simulink model "foc_signum_smo_g4"  (R2021b)
settings: Solver=FixedStepDiscrete  StartTime=0.0  StopTime=6  FixedStep=Tsw  RelTol=1e-3
undefined symbols (not defined in the file): a, B, b, current_ki, current_kp, DiscIntNeverNeededParam, Ibase, id_ref, J, k1_sta, k2_sta, Ks, load_torque, Ls, qpll, Rs, sigmoid_a, speed_ki, speed_kp, Ts_speed, Tsw, Vbase, Vdc, wbase
libraries: mcbcontrolslib x6, mcbplantlib x1, autolibpmsmexterior x1, simulink_extras x1
settings Model: Creator=gary  LastModifiedBy=gary
settings DebuggingCC: SFMachineParentedDataDiag=warning

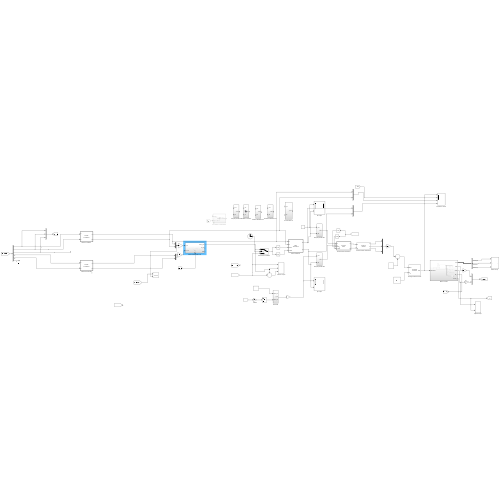
[thumbnail: Simulink's stored preview of the top-level diagram]
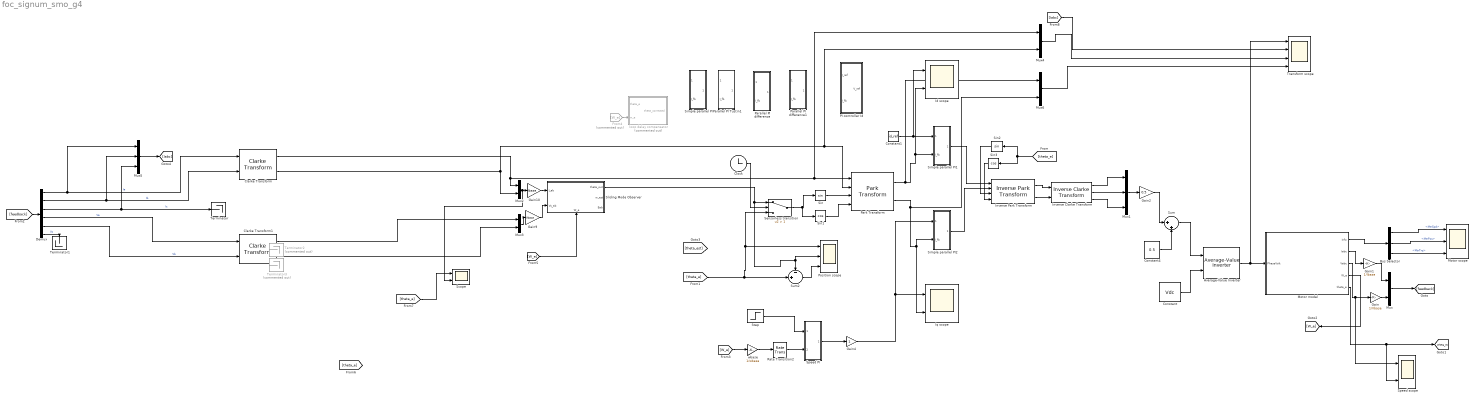
== system foc_signum_smo_g4 ==
  Average-Value Inverter : mcbplantlib/Average-Value Inverter
  Bus Selector : BusSelector  OutputSignals=MtrSpd,MtrPos,MtrTrq
  Clarke Transform : mcbcontrolslib/Clarke Transform  VariantControl=Variant2
  Clarke Transform1 : mcbcontrolslib/Clarke Transform  VariantControl=Variant2
  Clock : Clock
  Constant : Constant  Value=Vdc
  Constant1 : Constant  Value=id_ref
  Constant4 : Constant  Value=0.5
  Demux : Demux  Outputs=6
  From4 : From  Commented=on  GotoTag=W_e
  Gain : Gain  Gain=1/Vbase
  Gain1 : Gain  Gain=1/Ibase
  Gain10 : Gain  Gain=Ibase
  Gain2 : Gain  Gain=0.5
  Gain4 : Gain
  Gain9 : Gain  Gain=Vbase
  Id scope : Scope  NumInputPorts=2
  Inverse Clarke Transform : mcbcontrolslib/Inverse Clarke Transform
      settings: SourceProductBaseCode=MT
  Inverse Park Transform : mcbcontrolslib/Inverse Park Transform  AxisAlignment=D-axis
  Iq scope : Scope  NumInputPorts=2
  Motor model : Subsystem
  Motor scope : Scope  NumInputPorts=3
  Mux{,2..4,6} (5 alike) : Mux  Inputs=2
  Mux1 : Mux  Inputs=3
  Mux5 : Mux  Inputs=3
  PI controller Id : Subsystem
  Parallel PI Tustin1 : Subsystem
  Parallel PI difference : Subsystem
  Parallel PI difference1 : Subsystem
  Park Transform : mcbcontrolslib/Park Transform  AxisAlignment=D-axis
      settings: SourceProductBaseCode=MT
  Position scope : Scope  NumInputPorts=3
  Rate Transition2 : RateTransition  OutPortSampleTime=Ts_speed
  Scope : Scope  NumInputPorts=2
  Sensorless transition : Switch  Criteria=u2 > Threshold  Threshold=1
  Simple parallel PI : Subsystem
  Simple parallel PI1 : Subsystem
  Simple parallel PI2 : Subsystem
  Sin : Trigonometry
  Sin1 : Trigonometry  Operator=cos
  Sin2 : Trigonometry
  Sin3 : Trigonometry  Operator=cos
  Sliding Mode Observer : Subsystem
      settings: PortSchema="{\"entries\":[{\"content\":{\"sides\":[{\"content\":{\"connectorIds\":[\"In1\",\"In2\"]},\"type\":\"ConnectorPlacement.EquallySpacedRectSide\",\"uuid\":\"577b0a5e-906f-48ed-8129-dbceeacd07ca\"},{\"content\":{\"connectorIds\":[\"Out1\",\"Out2\",\"Out3\"],\"side\":\"RIGHT\"},\"type\":\"ConnectorPlacement.EquallySpacedRectSide\",\"uuid\":\"748cd512-9e16-4867-9350-2ceae49fd380\"},{\"content\":{\"connectorIds\":[],\"side\":\"TOP\"},\"type\":\"ConnectorPlacement.EquallySpacedRectSide\",\"uuid\":\"9a069db4-944b-4d2f-847d-3587eda2386e\"},{\"content\":{\"connectorIds\":[\"In3\"],\"side\":\"BOTTOM\"},\"type\":\"ConnectorPlacement.EquallySpacedRectSide\",\"uuid\":\"f06943a4-3386-47cc-a738-6805519a12d9\"}]},\"type\":\"ConnectorPlacement.EquallySpacedConnector\",\"uuid\":\"48fa9e95-782d-48ca-a522-50122ca51ecb\"}],\"packageUris\":[\"http://schema.mathworks.com/mf0/Connector/R2020b\"],\"version\":\"1.0\"}"
  Speed PI : Subsystem
  Speed scope : Scope  NumInputPorts=2
  Step : Step  Time=3  Before=0.25  After=0.5  SampleTime=0
  Sum : Sum  Inputs=|++
  Sum2 : Sum  Inputs=-+|
  Terminator : Terminator
  Terminator1 : Terminator
  Terminator2 : Terminator  Commented=on
  Terminator3 : Terminator  Commented=on
  Transform scope : Scope  NumInputPorts=4
  loop delay compensator : Subsystem  Commented=on
  wbase : Gain  Gain=1/wbase
  wires:
  Constant/1 -> Average-Value Inverter/2
  Motor model/1(Info) -> Bus Selector/1
  Bus Selector/2 -> Motor scope/2  "<MtrPos>"
  Bus Selector/3 -> Motor scope/3  "<MtrTrq>"
  Mux/1 -> [feedback]
  [feedback] -> Demux/1
  Demux/3 -> Mux5/3, Terminator/1  "Ic"
  Demux/1 -> Mux5/1, Clarke Transform/1  "Ia"
  Demux/2 -> Mux5/2, Clarke Transform/2  "Ib"
  Park Transform/1 -> Simple parallel PI1/2(I_fb), Id scope/2, Mux6/1
  Park Transform/2 -> Mux6/2, Simple parallel PI2/2(I_fb), Iq scope/2
  Constant1/1 -> Simple parallel PI1/1(I_ref), Id scope/1
  Simple parallel PI1/1(Vref) -> Inverse Park Transform/1
  Simple parallel PI2/1(Vref) -> Inverse Park Transform/2
  Inverse Park Transform/1 -> Inverse Clarke Transform/1
  Inverse Park Transform/2 -> Inverse Clarke Transform/2
  Inverse Clarke Transform/2 -> Mux1/2
  Inverse Clarke Transform/3 -> Mux1/3
  Inverse Clarke Transform/1 -> Mux1/1
  Motor model/2(Iabc) -> Gain1/1
  Gain1/1 -> Mux/1
  Motor model/3(Vabc) -> Speed scope/1, Gain/1
  Demux/6 -> Terminator1/1  "Vc"
  Clarke Transform/1 -> Mux2/1, Mux4/1, Park Transform/1
  Clarke Transform/2 -> Mux2/2, Mux4/2, Park Transform/2
  Sin/1 -> Park Transform/3
  Sin1/1 -> Park Transform/4
  Gain/1 -> Mux/2
  Mux1/1 -> Gain2/1
  Gain2/1 -> Sum/1
  Sum/1 -> Average-Value Inverter/1
  Constant4/1 -> Sum/2
  [theta_e] -> Position scope/1, Sensorless transition/3, Sum2/2
  Bus Selector/1 -> Motor scope/1  "<MtrSpd>"
  Clock/1 -> Sensorless transition/2
  Sliding Mode Observer/1(theta_out) -> Sum2/1, Position scope/2, Sensorless transition/1
  [W_e] -> wbase/1
  Step/1 -> Speed PI/1(Speed_ref)
  Rate Transition2/1 -> Speed PI/2(Speed_fb)
  Speed PI/1(I_ref) -> Gain4/1
  wbase/1 -> Rate Transition2/1
  Motor model/4(W_e) -> [W_e]
  Gain4/1 -> Simple parallel PI2/1(I_ref), Iq scope/1
  Demux/4 -> Clarke Transform1/1  "Va"
  Demux/5 -> Clarke Transform1/2  "Vb"
  Mux2/1 -> Scope/2, Gain10/1
  Gain10/1 -> Sliding Mode Observer/1(I_ab)
  Mux3/1 -> Gain9/1
  Gain9/1 -> Sliding Mode Observer/2(Vs_ab)
  Sum2/1 -> Position scope/3
  Clarke Transform1/1 -> Mux3/1
  Clarke Transform1/2 -> Mux3/2
  Average-Value Inverter/1 -> Transform scope/1, Motor model/1(PhaseVolt)
  From4/1 -> loop delay compensator/2(w_e)
  Sin2/1 -> Inverse Park Transform/3
  Sin3/1 -> Inverse Park Transform/4
  [theta_e] -> Sin2/1, Sin3/1
  Mux4/1 -> Transform scope/3
  Mux6/1 -> Transform scope/4
  Mux5/1 -> [Iabc]
  [Iabc] -> Transform scope/2
  [W_e] -> Sliding Mode Observer/3(W_e)
  Sensorless transition/1 -> Sin1/1, Sin/1
  Motor model/5(theta_e) -> Speed scope/2, [theta_e]
  [theta_e] -> Scope/1

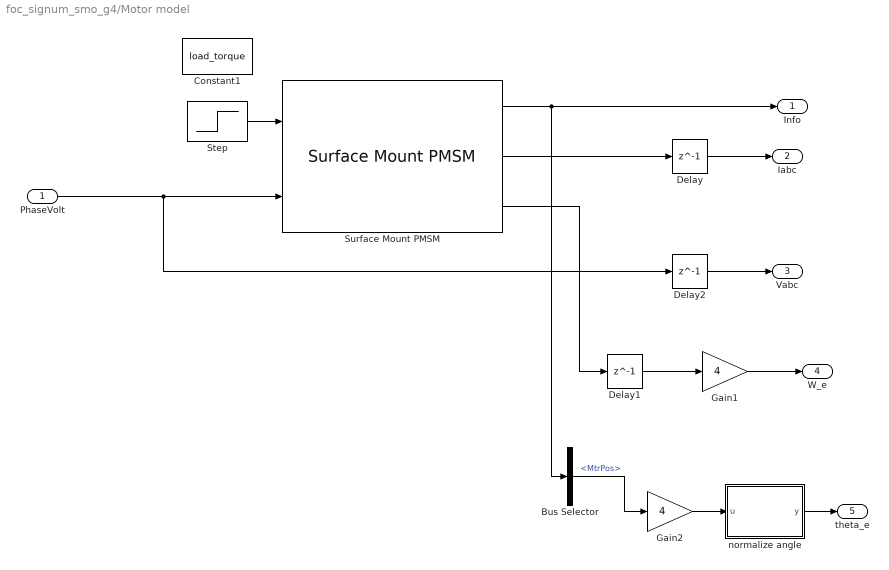
== system foc_signum_smo_g4/Motor model ==
  PhaseVolt : Inport
  Bus Selector : BusSelector  OutputSignals=MtrPos
  Constant1 : Constant  Value=load_torque
  Delay : Delay  DelayLength=1  InitialCondition=0
  Delay1 : Delay  DelayLength=1  InitialCondition=0
  Delay2 : Delay  DelayLength=1  InitialCondition=0
  Gain1 : Gain  Gain=4
  Gain2 : Gain  Gain=4
  Step : Step  Time=4  Before=-0.2  After=-0.4  SampleTime=0
  Surface Mount PMSM : autolibpmsmexterior/Surface Mount PMSM  port_config=Torque  sim_type=Discrete  Ts=Tsw  P=4  Rs=1.5*Rs  Ldq_=2*Ls  KConstText=Permanent flux linkage constant (lambda_pm):  lambda_pm=lambda  Ke=159.9771  Kt=1.323  mechanical=[J, B, 0]  idq0=[0 0]  theta_init=0  omega_init=150  KConst=lambda  lambda_pm_calc=lambda  RefBlkName='autolibpmsmexterior/Surface Mount PMSM'  aMode=5  Ldq="[0.0017      0.0017]"
      settings: SourceProductBaseCode=PW,DR,MT,UV,VE
  normalize angle : MATLAB Function  TreatAsAtomicUnit=on
  Info : Outport
  Iabc : Outport  Port=2
  Vabc : Outport  Port=3
  W_e : Outport  Port=4
  theta_e : Outport  Port=5
  wires:
  Surface Mount PMSM/1 -> Info/1, Bus Selector/1
  Surface Mount PMSM/2 -> Delay/1
  PhaseVolt/1 -> Delay2/1, Surface Mount PMSM/2
  Step/1 -> Surface Mount PMSM/1
  Surface Mount PMSM/3 -> Delay1/1
  Delay/1 -> Iabc/1
  Bus Selector/1 -> Gain2/1  "<MtrPos>"
  Delay1/1 -> Gain1/1
  Gain1/1 -> W_e/1
  Delay2/1 -> Vabc/1
  Gain2/1 -> normalize angle/1(u)
  normalize angle/1(y) -> theta_e/1

== system foc_signum_smo_g4/PI controller Id ==
  I_ref : Inport
  I_fb : Inport  Port=2
  Constant1 : Constant  Value=0
  Constant2 : Constant  Value=current_kp
  Constant3 : Constant  Value=current_ki*Tsw
  Constant4 : Constant  Value=0
  Discrete PI Controller with anti-windup & reset : mcbcontrolslib/Discrete PI Controller  with anti-windup & reset  UpperSaturationLimit=1  LowerSaturationLimit=-1
      settings: SourceProductBaseCode=MT
  Sum : Sum  Inputs=|+-
  V_ref : Outport
  wires:
  I_ref/1 -> Sum/1
  Constant4/1 -> Discrete PI Controller with anti-windup & reset/5
  Discrete PI Controller with anti-windup & reset/1 -> V_ref/1
  Constant1/1 -> Discrete PI Controller with anti-windup & reset/4
  I_fb/1 -> Sum/2
  Constant2/1 -> Discrete PI Controller with anti-windup & reset/2
  Sum/1 -> Discrete PI Controller with anti-windup & reset/1
  Constant3/1 -> Discrete PI Controller with anti-windup & reset/3

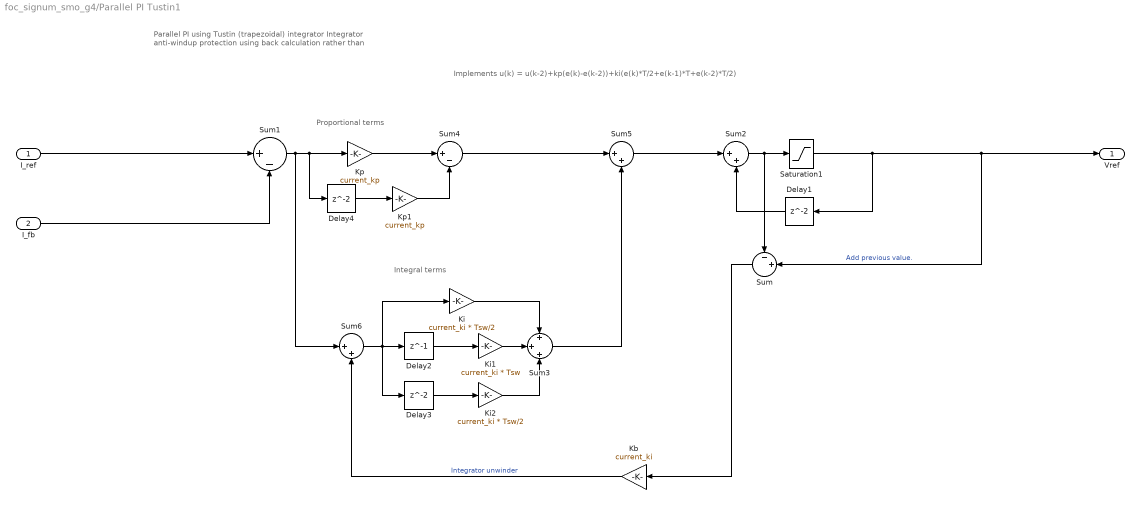
== system foc_signum_smo_g4/Parallel PI Tustin1 ==
  note: Implements u(k) = u(k-2)+kp(e(k)-e(k-2))+ki(e(k)*T/2+e(k-1)*T+e(k-2)*T/2)
  note: Integral terms
  note: Proportional terms
  note: Parallel PI using Tustin (trapezoidal) integrator
      | Integrator anti-windup protection using back calculation
      | rather than
  I_ref : Inport
  I_fb : Inport  Port=2
  Delay1 : Delay  InitialCondition=0
  Delay2 : Delay  DelayLength=1  InitialCondition=0
  Delay3 : Delay  InitialCondition=0
  Delay4 : Delay  InitialCondition=0
  Kb : Gain  Gain=current_ki
  Ki : Gain  Gain=current_ki * Tsw/2
  Ki1 : Gain  Gain=current_ki * Tsw
  Ki2 : Gain  Gain=current_ki * Tsw/2
  Kp : Gain  Gain=current_kp
  Kp1 : Gain  Gain=current_kp
  Saturation1 : Saturate  UpperLimit=1  LowerLimit=-1
  Sum : Sum  Inputs=-+|
  Sum1 : Sum  Inputs=|+-
  Sum2 : Sum  Inputs=|++
  Sum3 : Sum  Inputs=+|+|+
  Sum4 : Sum  Inputs=|+-
  Sum5 : Sum  Inputs=|++
  Sum6 : Sum  Inputs=|++
  Vref : Outport
  wires:
  Sum1/1 -> Sum6/1, Delay4/1, Kp/1
  I_fb/1 -> Sum1/2
  I_ref/1 -> Sum1/1
  Kp/1 -> Sum4/1
  Delay1/1 -> Sum2/2
  Sum2/1 -> Sum/1, Saturation1/1
  Sum/1 -> Kb/1
  Delay2/1 -> Ki1/1
  Delay3/1 -> Ki2/1
  Delay4/1 -> Kp1/1
  Kp1/1 -> Sum4/2
  Ki1/1 -> Sum3/2
  Ki/1 -> Sum3/1
  Ki2/1 -> Sum3/3
  Sum4/1 -> Sum5/1
  Sum6/1 -> Delay3/1, Delay2/1, Ki/1
  Sum3/1 -> Sum5/2
  Sum5/1 -> Sum2/1
  Kb/1 -> Sum6/2  "Integrator unwinder"
  Saturation1/1 -> Sum/2, Vref/1, Delay1/1  "Add previous value."

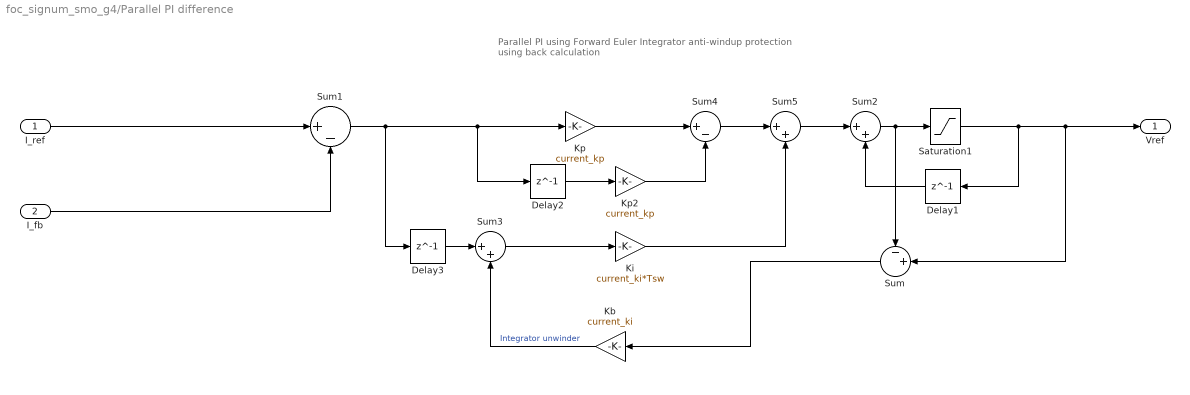
== system foc_signum_smo_g4/Parallel PI difference ==
  note: Parallel PI using Forward Euler
      | Integrator anti-windup protection using back calculation
  I_ref : Inport
  I_fb : Inport  Port=2
  Delay1 : Delay  DelayLength=1  InitialCondition=0
  Delay2 : Delay  DelayLength=1  InitialCondition=0
  Delay3 : Delay  DelayLength=1  InitialCondition=0
  Kb : Gain  Gain=current_ki
  Ki : Gain  Gain=current_ki*Tsw
  Kp : Gain  Gain=current_kp
  Kp2 : Gain  Gain=current_kp
  Saturation1 : Saturate  UpperLimit=1  LowerLimit=0
  Sum : Sum  Inputs=-+|
  Sum1 : Sum  Inputs=|+-
  Sum2 : Sum  Inputs=|++
  Sum3 : Sum  Inputs=|++
  Sum4 : Sum  Inputs=|+-
  Sum5 : Sum  Inputs=|++
  Vref : Outport
  wires:
  I_fb/1 -> Sum1/2
  I_ref/1 -> Sum1/1
  Sum1/1 -> Delay2/1, Kp/1, Delay3/1
  Kp/1 -> Sum4/1
  Delay1/1 -> Sum2/2
  Sum2/1 -> Saturation1/1, Sum/1
  Saturation1/1 -> Sum/2, Vref/1, Delay1/1
  Kb/1 -> Sum3/2  "Integrator unwinder"
  Sum/1 -> Kb/1
  Delay2/1 -> Kp2/1
  Kp2/1 -> Sum4/2
  Sum3/1 -> Ki/1
  Delay3/1 -> Sum3/1
  Sum4/1 -> Sum5/1
  Ki/1 -> Sum5/2
  Sum5/1 -> Sum2/1

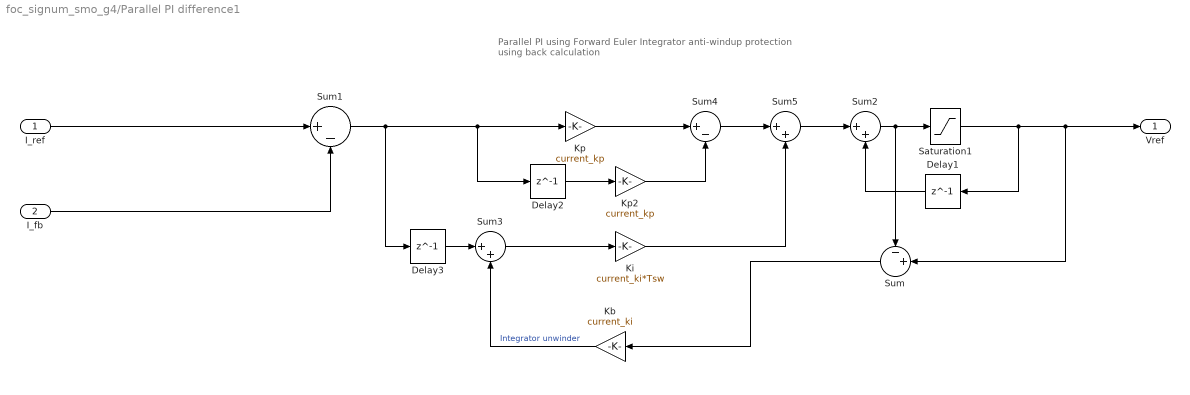
== system foc_signum_smo_g4/Parallel PI difference1 ==
  note: Parallel PI using Forward Euler
      | Integrator anti-windup protection using back calculation
  I_ref : Inport
  I_fb : Inport  Port=2
  Delay1 : Delay  DelayLength=1  InitialCondition=0
  Delay2 : Delay  DelayLength=1  InitialCondition=0
  Delay3 : Delay  DelayLength=1  InitialCondition=0
  Kb : Gain  Gain=current_ki
  Ki : Gain  Gain=current_ki*Tsw
  Kp : Gain  Gain=current_kp
  Kp2 : Gain  Gain=current_kp
  Saturation1 : Saturate  UpperLimit=1  LowerLimit=0
  Sum : Sum  Inputs=-+|
  Sum1 : Sum  Inputs=|+-
  Sum2 : Sum  Inputs=|++
  Sum3 : Sum  Inputs=|++
  Sum4 : Sum  Inputs=|+-
  Sum5 : Sum  Inputs=|++
  Vref : Outport
  wires:
  I_fb/1 -> Sum1/2
  I_ref/1 -> Sum1/1
  Sum1/1 -> Delay2/1, Kp/1, Delay3/1
  Kp/1 -> Sum4/1
  Delay1/1 -> Sum2/2
  Sum2/1 -> Saturation1/1, Sum/1
  Saturation1/1 -> Sum/2, Vref/1, Delay1/1
  Kb/1 -> Sum3/2  "Integrator unwinder"
  Sum/1 -> Kb/1
  Delay2/1 -> Kp2/1
  Kp2/1 -> Sum4/2
  Sum3/1 -> Ki/1
  Delay3/1 -> Sum3/1
  Sum4/1 -> Sum5/1
  Ki/1 -> Sum5/2
  Sum5/1 -> Sum2/1

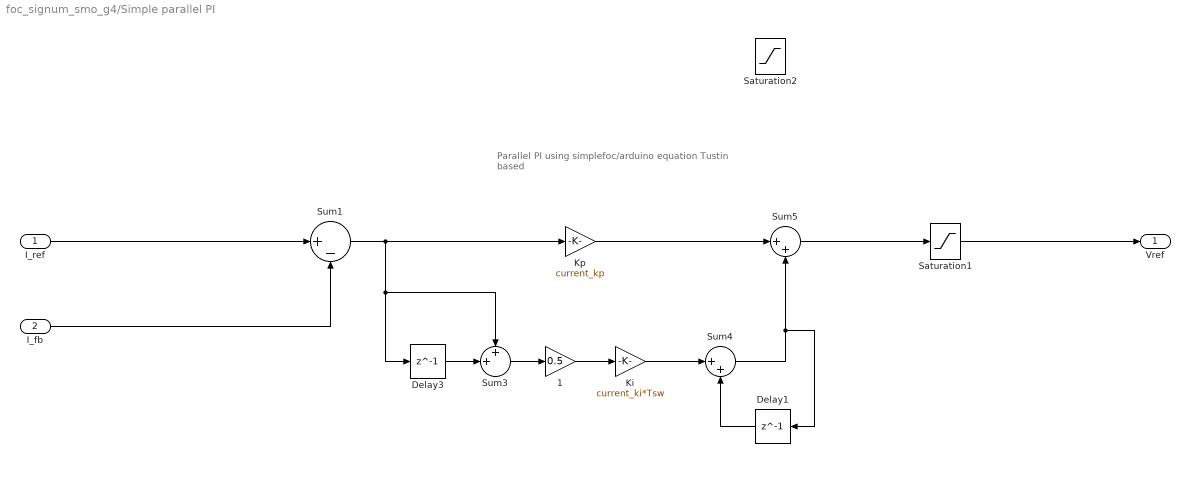
== system foc_signum_smo_g4/Simple parallel PI ==
  note: Parallel PI using simplefoc/arduino equation
      | Tustin based
  I_ref : Inport
  I_fb : Inport  Port=2
  1 : Gain  Gain=0.5
  Delay1 : Delay  DelayLength=1  InitialCondition=0
  Delay3 : Delay  DelayLength=1  InitialCondition=0
  Ki : Gain  Gain=current_ki*Tsw
  Kp : Gain  Gain=current_kp
  Saturation1 : Saturate  UpperLimit=1  LowerLimit=0
  Saturation2 : Saturate  UpperLimit=1  LowerLimit=0
  Sum1 : Sum  Inputs=|+-
  Sum3 : Sum  Inputs=++|
  Sum4 : Sum  Inputs=|++
  Sum5 : Sum  Inputs=|++
  Vref : Outport
  wires:
  I_fb/1 -> Sum1/2
  I_ref/1 -> Sum1/1
  Sum5/1 -> Saturation1/1
  Saturation1/1 -> Vref/1
  Sum3/1 -> 1/1
  Kp/1 -> Sum5/1
  Delay3/1 -> Sum3/2
  Sum1/1 -> Kp/1, Sum3/1, Delay3/1
  1/1 -> Ki/1
  Ki/1 -> Sum4/1
  Sum4/1 -> Delay1/1, Sum5/2
  Delay1/1 -> Sum4/2

== system foc_signum_smo_g4/Simple parallel PI1 ==
  note: Parallel PI using simplefoc/arduino equation
      | Tustin based
  I_ref : Inport
  I_fb : Inport  Port=2
  1 : Gain  Gain=0.5
  Delay1 : Delay  DelayLength=1  InitialCondition=0
  Delay3 : Delay  DelayLength=1  InitialCondition=0
  Ki : Gain  Gain=current_ki*Tsw
  Kp : Gain  Gain=current_kp
  Saturation1 : Saturate  UpperLimit=1  LowerLimit=-1
  Saturation2 : Saturate  UpperLimit=1  LowerLimit=0
  Sum1 : Sum  Inputs=|+-
  Sum3 : Sum  Inputs=++|
  Sum4 : Sum  Inputs=|++
  Sum5 : Sum  Inputs=|++
  Vref : Outport
  wires:
  I_fb/1 -> Sum1/2
  I_ref/1 -> Sum1/1
  Sum5/1 -> Saturation1/1
  Saturation1/1 -> Vref/1
  Sum3/1 -> 1/1
  Kp/1 -> Sum5/1
  Delay3/1 -> Sum3/2
  Sum1/1 -> Kp/1, Sum3/1, Delay3/1
  1/1 -> Ki/1
  Ki/1 -> Sum4/1
  Sum4/1 -> Delay1/1, Sum5/2
  Delay1/1 -> Sum4/2

== system foc_signum_smo_g4/Simple parallel PI2 ==
  note: Parallel PI using simplefoc/arduino equation
      | Tustin based
  I_ref : Inport
  I_fb : Inport  Port=2
  1 : Gain  Gain=0.5
  Delay1 : Delay  DelayLength=1  InitialCondition=0
  Delay3 : Delay  DelayLength=1  InitialCondition=0
  Ki : Gain  Gain=current_ki*Tsw
  Kp : Gain  Gain=current_kp
  Saturation1 : Saturate  UpperLimit=1  LowerLimit=-1
  Saturation2 : Saturate  UpperLimit=1  LowerLimit=0
  Sum1 : Sum  Inputs=|+-
  Sum3 : Sum  Inputs=++|
  Sum4 : Sum  Inputs=|++
  Sum5 : Sum  Inputs=|++
  Vref : Outport
  wires:
  I_fb/1 -> Sum1/2
  I_ref/1 -> Sum1/1
  Sum5/1 -> Saturation1/1
  Saturation1/1 -> Vref/1
  Sum3/1 -> 1/1
  Kp/1 -> Sum5/1
  Delay3/1 -> Sum3/2
  Sum1/1 -> Kp/1, Sum3/1, Delay3/1
  1/1 -> Ki/1
  Ki/1 -> Sum4/1
  Sum4/1 -> Delay1/1, Sum5/2
  Delay1/1 -> Sum4/2

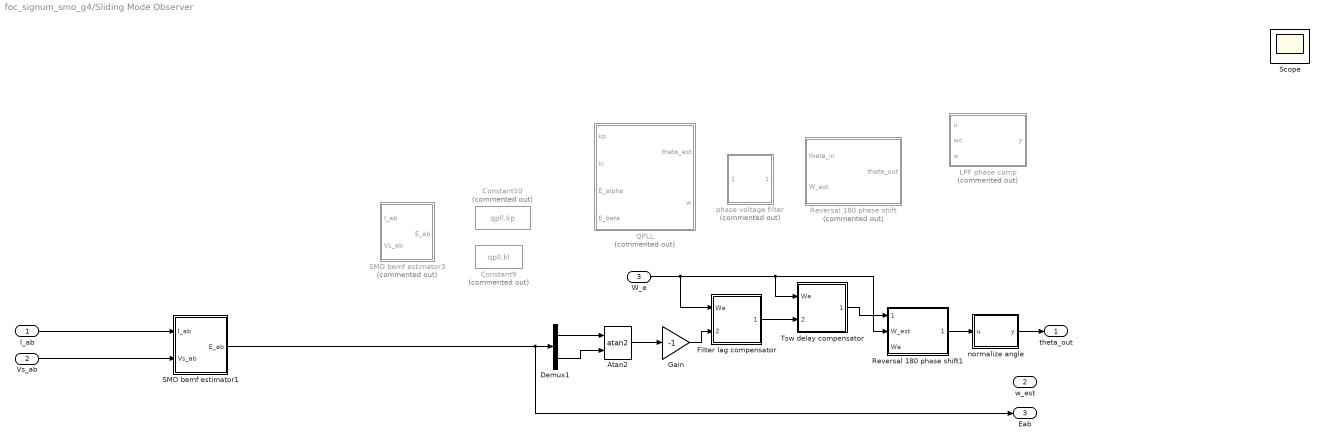
== system foc_signum_smo_g4/Sliding Mode Observer ==
  I_ab : Inport
  Vs_ab : Inport  Port=2
  W_e : Inport  Port=3
  Atan2 : Trigonometry  Operator=atan2
  Constant10 : Constant  Commented=on  Value=qpll.kp
  Constant9 : Constant  Commented=on  Value=qpll.ki
  Demux1 : Demux  Outputs=2
  Filter lag compensator : Subsystem
  Gain : Gain  Gain=-1
  LPF phase comp : MATLAB Function  Commented=on  TreatAsAtomicUnit=on
  QPLL : Subsystem  Commented=on
  Reversal 180 phase shift : Subsystem  Commented=on
  Reversal 180 phase shift1 : Subsystem
      settings: PortSchema="{\"entries\":[{\"content\":{\"sides\":[{\"content\":{\"connectorIds\":[\"In1\",\"In2\",\"Out2\"]},\"type\":\"ConnectorPlacement.EquallySpacedRectSide\",\"uuid\":\"bee660c5-5095-4afe-927e-ee79dc421287\"},{\"content\":{\"connectorIds\":[\"Out1\"],\"side\":\"RIGHT\"},\"type\":\"ConnectorPlacement.EquallySpacedRectSide\",\"uuid\":\"50128ad2-9f3e-46fb-af5a-e60f178d5f38\"},{\"content\":{\"connectorIds\":[],\"side\":\"TOP\"},\"type\":\"ConnectorPlacement.EquallySpacedRectSide\",\"uuid\":\"e659ec01-5289-4ab3-890a-571c274b67fc\"}]},\"type\":\"ConnectorPlacement.EquallySpacedConnector\",\"uuid\":\"95e6addf-8d53-4528-81dc-23509886194a\"}],\"packageUris\":[\"http://schema.mathworks.com/mf0/Connector/R2020b\"],\"version\":\"1.0\"}"
  SMO bemf estimator1 : Subsystem
  SMO bemf estimator3 : Subsystem  Commented=on
  Scope : Scope  NumInputPorts=2
  Tsw delay compensator : Subsystem
  normalize angle : MATLAB Function  TreatAsAtomicUnit=on
  phase voltage filter : Subsystem  Commented=on
  theta_out : Outport
  w_est : Outport  Port=2
  Eab : Outport  Port=3
  wires:
  Vs_ab/1 -> SMO bemf estimator1/2(Vs_ab)
  I_ab/1 -> SMO bemf estimator1/1(I_ab)
  SMO bemf estimator1/1(E_ab) -> Eab/1, Demux1/1
  Atan2/1 -> Gain/1
  Reversal 180 phase shift1/1(theta_out) -> normalize angle/1(u)
  normalize angle/1(y) -> theta_out/1
  Demux1/1 -> Atan2/1
  Demux1/2 -> Atan2/2
  Gain/1 -> Filter lag compensator/2(Theta)
  Filter lag compensator/1(Theta_out) -> Tsw delay compensator/2(Theta)
  Tsw delay compensator/1(Theta_out) -> Reversal 180 phase shift1/1(theta_in)
  W_e/1 -> Filter lag compensator/1(We), Reversal 180 phase shift1/2(W_est), Tsw delay compensator/1(We)

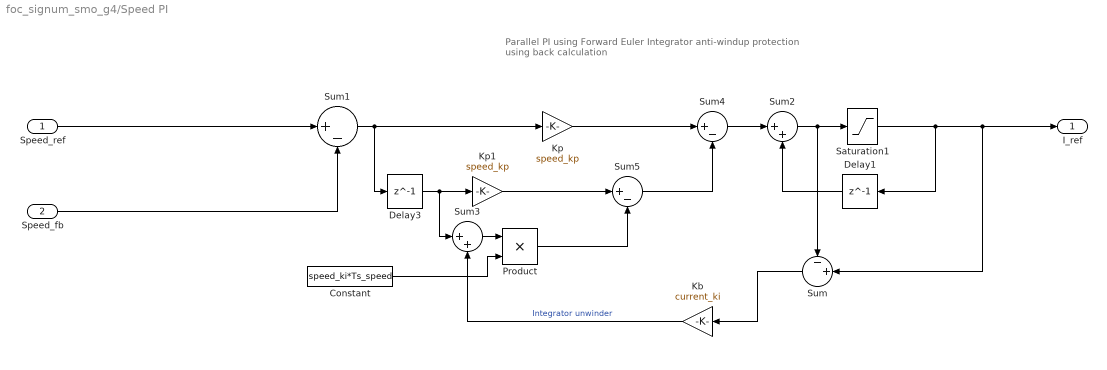
== system foc_signum_smo_g4/Speed PI ==
  note: Parallel PI using Forward Euler
      | Integrator anti-windup protection using back calculation
  Speed_ref : Inport
  Speed_fb : Inport  Port=2
  Constant : Constant  Value=speed_ki*Ts_speed
  Delay1 : Delay  DelayLength=1  InitialCondition=0
  Delay3 : Delay  DelayLength=1  InitialCondition=0
  Kb : Gain  Gain=current_ki
  Kp : Gain  Gain=speed_kp
  Kp1 : Gain  Gain=speed_kp
  Product : Product
  Saturation1 : Saturate  UpperLimit=1  LowerLimit=-1
  Sum : Sum  Inputs=-+|
  Sum1 : Sum  Inputs=|+-
  Sum2 : Sum  Inputs=|++
  Sum3 : Sum  Inputs=|++
  Sum4 : Sum  Inputs=|+-
  Sum5 : Sum  Inputs=|+-
  I_ref : Outport
  wires:
  Sum1/1 -> Delay3/1, Kp/1
  Speed_fb/1 -> Sum1/2
  Speed_ref/1 -> Sum1/1
  Constant/1 -> Product/2
  Delay3/1 -> Kp1/1, Sum3/1
  Kp1/1 -> Sum5/1
  Kp/1 -> Sum4/1
  Delay1/1 -> Sum2/2
  Sum4/1 -> Sum2/1
  Sum2/1 -> Sum/1, Saturation1/1
  Sum5/1 -> Sum4/2
  Product/1 -> Sum5/2
  Sum3/1 -> Product/1
  Kb/1 -> Sum3/2  "Integrator unwinder"
  Sum/1 -> Kb/1
  Saturation1/1 -> Sum/2, I_ref/1, Delay1/1

== system foc_signum_smo_g4/loop delay compensator ==
  note: Compensate for discrete delay of control loop.
      | Advance angle by the amount rotated in Tsw
  theta_e : Inport
  w_e : Inport  Port=2
  Gain6 : Gain  Gain=Tsw
  Sum3 : Sum  Inputs=|++
  theta_corrected : Outport
  wires:
  w_e/1 -> Gain6/1
  theta_e/1 -> Sum3/1
  Gain6/1 -> Sum3/2
  Sum3/1 -> theta_corrected/1

== system foc_signum_smo_g4/Sliding Mode Observer/Filter lag compensator ==
  We : Inport
  Theta : Inport  Port=2
  Divide : Product  Inputs=*/
  Gain1 : Gain
  Sum : Sum  Inputs=++|
  we at 1rad phase lag : Constant  Value=4850
  Theta_out : Outport
  wires:
  we at 1rad phase lag/1 -> Divide/2
  We/1 -> Divide/1
  Gain1/1 -> Sum/1
  Theta/1 -> Sum/2
  Divide/1 -> Gain1/1
  Sum/1 -> Theta_out/1

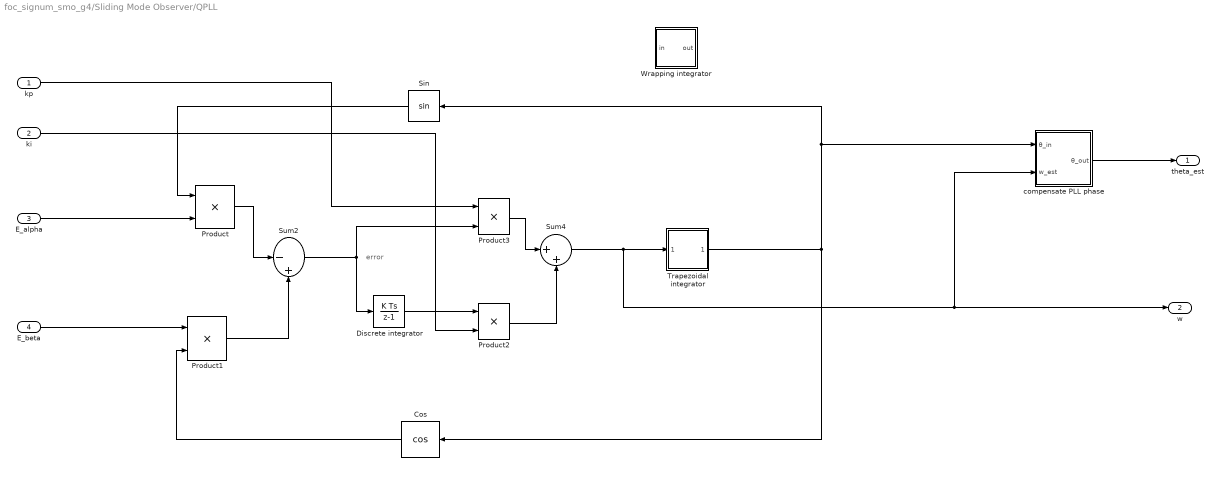
== system foc_signum_smo_g4/Sliding Mode Observer/QPLL ==
  note: error
  kp : Inport
  ki : Inport  Port=2
  E_alpha : Inport  Port=3
  E_beta : Inport  Port=4
  Cos : Trigonometry  Operator=cos
  Discrete integrator : DiscreteIntegrator  SampleTime=-1  ICPrevOutput=DiscIntNeverNeededParam  ICPrevScaledInput=DiscIntNeverNeededParam
  Product{,1..3} (4 alike) : Product
  Sin : Trigonometry
  Sum2 : Sum  Inputs=|-+
  Sum4 : Sum  Inputs=|++
  Trapezoidal integrator : Subsystem
  Wrapping integrator : Subsystem
      mask help: The integrator uses the Forward Euler method and wraps its state between 0 and 2*pi.
  compensate PLL phase : Subsystem
  theta_est : Outport
  w : Outport  Port=2
  wires:
  Sin/1 -> Product/1
  Cos/1 -> Product1/2
  Sum4/1 -> Trapezoidal integrator/1(Input), compensate PLL phase/2(w_est), w/1
  Product1/1 -> Sum2/2
  Product/1 -> Sum2/1
  kp/1 -> Product3/1
  Discrete integrator/1 -> Product2/1
  ki/1 -> Product2/2
  Product3/1 -> Sum4/1
  Product2/1 -> Sum4/2
  compensate PLL phase/1(θ_out) -> theta_est/1
  E_alpha/1 -> Product/2
  E_beta/1 -> Product1/1
  Trapezoidal integrator/1(Output) -> Cos/1, Sin/1, compensate PLL phase/1(θ_in)
  Sum2/1 -> Discrete integrator/1, Product3/2

== system foc_signum_smo_g4/Sliding Mode Observer/Reversal 180 phase shift ==
  theta_in : Inport
  W_est : Inport  Port=2
  Constant2 : Constant  Value=0
  Constant3 : Constant  Value=pi
  Constant4 : Constant  Value=2*pi
  Mod : Math  Operator=mod  SaturateOnIntegerOverflow=on
  Sign : Signum
  Sum : Sum  Inputs=|++
  Switch : Switch  Criteria=u2 > Threshold
  theta_out : Outport
  wires:
  Constant2/1 -> Switch/1
  Constant3/1 -> Switch/3
  Sum/1 -> Mod/1
  Constant4/1 -> Mod/2
  Switch/1 -> Sum/1
  Sign/1 -> Switch/2
  Mod/1 -> theta_out/1
  theta_in/1 -> Sum/2
  W_est/1 -> Sign/1

== system foc_signum_smo_g4/Sliding Mode Observer/Reversal 180 phase shift1 ==
  theta_in : Inport
  W_est : Inport  Port=2
  Constant2 : Constant  Value=0
  Constant3 : Constant  Value=pi
  Sign : Signum
  Sum : Sum  Inputs=|++
  Switch : Switch  Criteria=u2 > Threshold
  theta_out : Outport
  We : Outport  Port=2
  wires:
  Constant2/1 -> Switch/1
  Constant3/1 -> Switch/3
  Switch/1 -> Sum/1
  Sign/1 -> Switch/2
  theta_in/1 -> Sum/2
  W_est/1 -> Sign/1
  Sum/1 -> theta_out/1

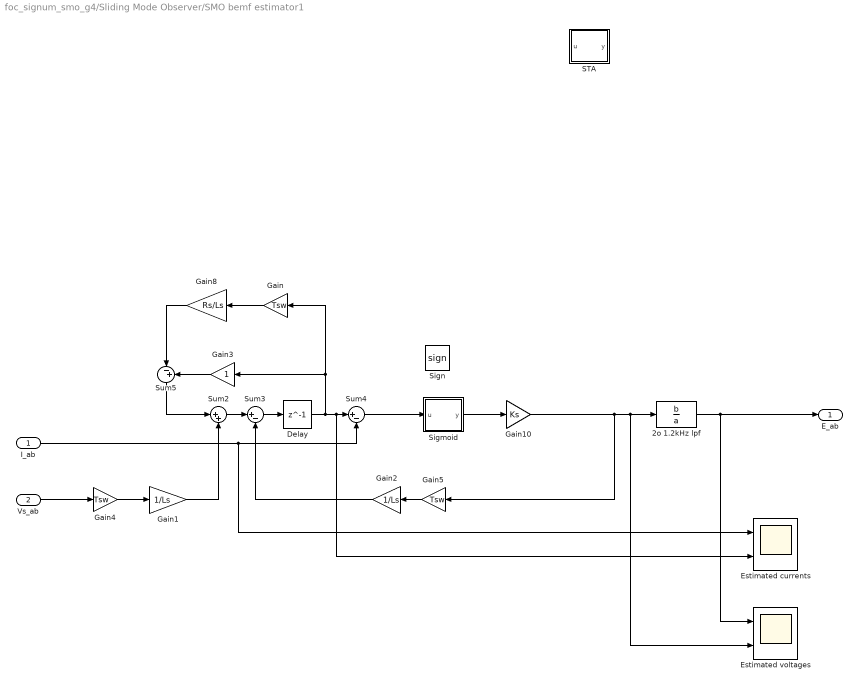
== system foc_signum_smo_g4/Sliding Mode Observer/SMO bemf estimator1 ==
  I_ab : Inport
  Vs_ab : Inport  Port=2
  2o 1.2kHz lpf : DiscreteFilter  Numerator=b  Denominator=a
  Delay : Delay  DelayLength=1  InitialCondition=0
  Estimated currents : Scope  NumInputPorts=2
  Estimated voltages : Scope  NumInputPorts=2
  Gain : Gain  Gain=Tsw
  Gain1 : Gain  Gain=1/Ls
  Gain10 : Gain  Gain=Ks
  Gain2 : Gain  Gain=1/Ls
  Gain3 : Gain
  Gain4 : Gain  Gain=Tsw
  Gain5 : Gain  Gain=Tsw
  Gain8 : Gain  Gain=Rs/Ls
  STA : Subsystem
      mask Display: plot(linspace(-1,1,100),(2./(1+exp(-10*linspace(-1,1,100))))-1)
  Sigmoid : Subsystem
      mask Display: plot(linspace(-1,1,100),(2./(1+exp(-10*linspace(-1,1,100))))-1)
  Sign : Signum
  Sum2 : Sum  Inputs=|++
  Sum3 : Sum  Inputs=|+-
  Sum4 : Sum  Inputs=|+-
  Sum5 : Sum  Inputs=|-+
  E_ab : Outport
  wires:
  Sum5/1 -> Sum2/1
  Gain8/1 -> Sum5/1
  Sum2/1 -> Sum3/1
  Sum3/1 -> Delay/1
  Vs_ab/1 -> Gain4/1
  I_ab/1 -> Estimated currents/1, Sum4/2
  Gain2/1 -> Sum3/2
  Gain/1 -> Gain8/1
  Gain5/1 -> Gain2/1
  Gain1/1 -> Sum2/2
  Gain4/1 -> Gain1/1
  Gain3/1 -> Sum5/2
  Delay/1 -> Gain3/1, Gain/1, Estimated currents/2, Sum4/1
  Sum4/1 -> Sigmoid/1(u)
  Sigmoid/1(y) -> Gain10/1
  Gain10/1 -> 2o 1.2kHz lpf/1, Estimated voltages/2, Gain5/1
  2o 1.2kHz lpf/1 -> E_ab/1, Estimated voltages/1

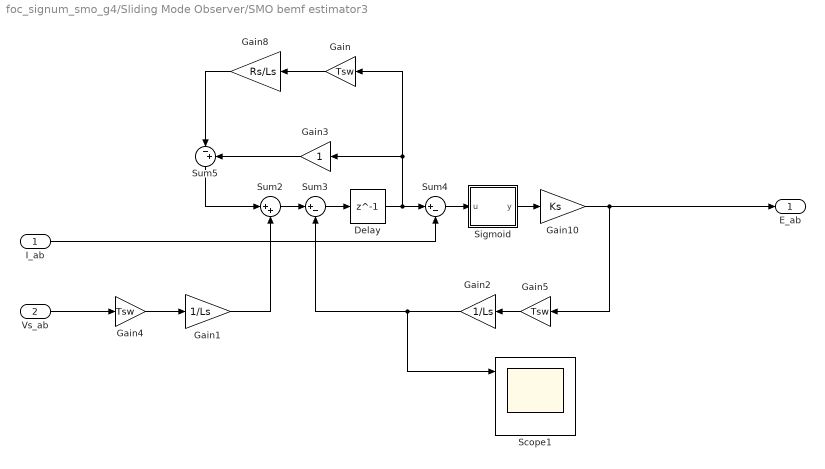
== system foc_signum_smo_g4/Sliding Mode Observer/SMO bemf estimator3 ==
  I_ab : Inport
  Vs_ab : Inport  Port=2
  Delay : Delay  DelayLength=1  InitialCondition=0
  Gain : Gain  Gain=Tsw
  Gain1 : Gain  Gain=1/Ls
  Gain10 : Gain  Gain=Ks
  Gain2 : Gain  Gain=1/Ls
  Gain3 : Gain
  Gain4 : Gain  Gain=Tsw
  Gain5 : Gain  Gain=Tsw
  Gain8 : Gain  Gain=Rs/Ls
  Scope1 : Scope  NumInputPorts=3
  Sigmoid : Subsystem
      mask Display: plot(linspace(-1,1,100),(2./(1+exp(-10*linspace(-1,1,100))))-1)
  Sum2 : Sum  Inputs=|++
  Sum3 : Sum  Inputs=|+-
  Sum4 : Sum  Inputs=|+-
  Sum5 : Sum  Inputs=|-+
  E_ab : Outport
  wires:
  Sum5/1 -> Sum2/1
  Gain8/1 -> Sum5/1
  Sum4/1 -> Sigmoid/1(u)
  Sum2/1 -> Sum3/1
  Sigmoid/1(y) -> Gain10/1
  Gain10/1 -> Gain5/1, E_ab/1
  Sum3/1 -> Delay/1
  Vs_ab/1 -> Gain4/1
  Delay/1 -> Gain/1, Gain3/1, Sum4/1
  I_ab/1 -> Sum4/2
  Gain2/1 -> Scope1/1, Sum3/2
  Gain/1 -> Gain8/1
  Gain5/1 -> Gain2/1
  Gain1/1 -> Sum2/2
  Gain4/1 -> Gain1/1
  Gain3/1 -> Sum5/2

== system foc_signum_smo_g4/Sliding Mode Observer/Tsw delay compensator ==
  We : Inport
  Theta : Inport  Port=2
  Gain1 : Gain  Gain=Tsw
  Sum : Sum  Inputs=++|
  Theta_out : Outport
  wires:
  We/1 -> Gain1/1
  Gain1/1 -> Sum/1
  Theta/1 -> Sum/2
  Sum/1 -> Theta_out/1

== system foc_signum_smo_g4/Sliding Mode Observer/phase voltage filter ==
  lpf in : Inport
  Instaspin lpf tf : simulink_extras/Additional Discrete/Discrete Transfer Fcn (with initial outputs)  N=[0.006918, 0.006659]  D=[1 -0.8919]  U0=[1]  Y0=0  TS=-1
      settings: SourceProductBaseCode=SL
  Rate Transition1 : RateTransition  OutPortSampleTime=Tsw
  lpf out : Outport
  wires:
  Rate Transition1/1 -> Instaspin lpf tf/1
  Instaspin lpf tf/1 -> lpf out/1
  lpf in/1 -> Rate Transition1/1

== system foc_signum_smo_g4/Sliding Mode Observer/QPLL/Trapezoidal integrator ==
  Input : Inport
  Delay1 : Delay  DelayLength=1
  Delay2 : Delay  DelayLength=1
  Gain : Gain  Gain=Tsw
  Gain1 : Gain  Gain=0.5
  Math Function : Math  Operator=mod  SignedPower=on  OutputSignalType=real  SaturateOnIntegerOverflow=on
  Sum1 : Sum  Inputs=|++
  Sum3 : Sum  Inputs=|++
  cst : Constant  Value=2*pi  OutDataTypeStr=Inherit: Inherit via back propagation
  Output : Outport
  wires:
  cst/1 -> Math Function/2
  Sum3/1 -> Gain1/1
  Gain/1 -> Sum1/1
  Input/1 -> Delay2/1, Sum3/1
  Delay2/1 -> Sum3/2
  Gain1/1 -> Gain/1
  Math Function/1 -> Output/1, Delay1/1
  Sum1/1 -> Math Function/1
  Delay1/1 -> Sum1/2

== system foc_signum_smo_g4/Sliding Mode Observer/QPLL/Wrapping integrator ==
  in : Inport
  Delay1 : Delay  DelayLength=1
  Gain : Gain  Gain=Tsw
  Math Function : Math  Operator=mod  SignedPower=on  OutputSignalType=real  SaturateOnIntegerOverflow=on
  Sum1 : Sum  Inputs=|++
  Weighted Sample Time : SampleTimeMath  TsampMathOp=*
  cst : Constant  Value=2*pi  OutDataTypeStr=Inherit: Inherit via back propagation
  out : Outport
  wires:
  in/1 -> Gain/1
  cst/1 -> Math Function/2
  Gain/1 -> Sum1/1
  Sum1/1 -> Math Function/1
  Delay1/1 -> Sum1/2
  Math Function/1 -> out/1, Delay1/1

== system foc_signum_smo_g4/Sliding Mode Observer/QPLL/compensate PLL phase ==
  θ_in : Inport
  w_est : Inport  Port=2
  Constant : Constant  Value=2*pi
  Gain : Gain  Gain=pi/2
  Mod : Math  Operator=mod  SaturateOnIntegerOverflow=on
  Sign : Signum
  Sum : Sum  Inputs=|++
  θ_out : Outport
  wires:
  θ_in/1 -> Sum/1
  Sign/1 -> Gain/1
  w_est/1 -> Sign/1
  Gain/1 -> Sum/2
  Sum/1 -> Mod/1
  Constant/1 -> Mod/2
  Mod/1 -> θ_out/1

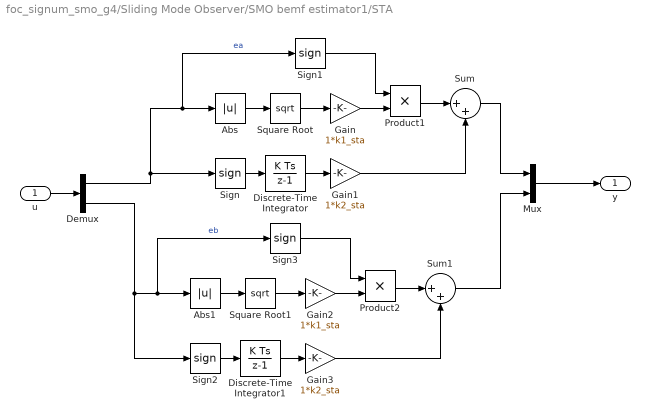
== system foc_signum_smo_g4/Sliding Mode Observer/SMO bemf estimator1/STA ==
  u : Inport
  Abs : Abs
  Abs1 : Abs
  Demux : Demux  Outputs=2
  Discrete-Time Integrator : DiscreteIntegrator  SampleTime=-1  ICPrevOutput=DiscIntNeverNeededParam  ICPrevScaledInput=DiscIntNeverNeededParam
  Discrete-Time Integrator1 : DiscreteIntegrator  SampleTime=-1  ICPrevOutput=DiscIntNeverNeededParam  ICPrevScaledInput=DiscIntNeverNeededParam
  Gain : Gain  Gain=1*k1_sta
  Gain1 : Gain  Gain=1*k2_sta
  Gain2 : Gain  Gain=1*k1_sta
  Gain3 : Gain  Gain=1*k2_sta
  Mux : Mux  Inputs=2
  Product1 : Product
  Product2 : Product
  Sign{,1..3} (4 alike) : Signum
  Square Root : Sqrt  SaturateOnIntegerOverflow=on
  Square Root1 : Sqrt  SaturateOnIntegerOverflow=on
  Sum : Sum  Inputs=|++
  Sum1 : Sum  Inputs=|++
  y : Outport
  wires:
  Square Root/1 -> Gain/1
  Gain/1 -> Product1/2
  Sign1/1 -> Product1/1
  Abs/1 -> Square Root/1
  Product1/1 -> Sum/1
  Sign/1 -> Discrete-Time Integrator/1
  Discrete-Time Integrator/1 -> Gain1/1
  Gain1/1 -> Sum/2
  Sum/1 -> Mux/1
  u/1 -> Demux/1
  Demux/1 -> Sign1/1, Abs/1, Sign/1  "ea"
  Mux/1 -> y/1
  Abs1/1 -> Square Root1/1
  Sign3/1 -> Product2/1
  Demux/2 -> Sign2/1, Sign3/1, Abs1/1  "eb"
  Product2/1 -> Sum1/1
  Gain3/1 -> Sum1/2
  Square Root1/1 -> Gain2/1
  Gain2/1 -> Product2/2
  Sum1/1 -> Mux/2
  Sign2/1 -> Discrete-Time Integrator1/1
  Discrete-Time Integrator1/1 -> Gain3/1

== system foc_signum_smo_g4/Sliding Mode Observer/SMO bemf estimator1/Sigmoid ==
  u : Inport
  Constant : Constant  Value=sigmoid_a
  Demux : Demux  Outputs=2
  Mux : Mux  Inputs=2
  sigmoid : MATLAB Function  TreatAsAtomicUnit=on
  sigmoid1 : MATLAB Function  TreatAsAtomicUnit=on
  y : Outport
  wires:
  Demux/2 -> sigmoid1/1(u)
  Demux/1 -> sigmoid/1(u)
  u/1 -> Demux/1
  sigmoid1/1(y) -> Mux/2
  sigmoid/1(y) -> Mux/1
  Mux/1 -> y/1
  Constant/1 -> sigmoid1/2(a), sigmoid/2(a)

== system foc_signum_smo_g4/Sliding Mode Observer/SMO bemf estimator3/Sigmoid ==
  u : Inport
  Constant : Constant  Value=sigmoid_a
  Demux : Demux  Outputs=2
  Mux : Mux  Inputs=2
  sigmoid : MATLAB Function  TreatAsAtomicUnit=on
  sigmoid1 : MATLAB Function  TreatAsAtomicUnit=on
  y : Outport
  wires:
  Demux/2 -> sigmoid1/1(u)
  Demux/1 -> sigmoid/1(u)
  u/1 -> Demux/1
  sigmoid1/1(y) -> Mux/2
  sigmoid/1(y) -> Mux/1
  Mux/1 -> y/1
  Constant/1 -> sigmoid1/2(a), sigmoid/2(a)

== matlab function foc_signum_smo_g4/Sliding Mode Observer/normalize angle ==
  data: u input; y output
function y = norm_angle(u)
% Normalize angle in radians to between -pi and pi using Matlab's
% wraptopi()

y = wrapToPi(u);

== matlab function foc_signum_smo_g4/Sliding Mode Observer/LPF phase comp ==
  data: u input; y output; wc input; w input
function y = phase_comp(u, wc, w)
% Compensate for first order low-pass filter attentuation
% Using gain = 1 / (sqrt(1+(w/wc).^2));
% Note pole frequency is wc

lag = atan(w/wc);
y = u + lag;
%y = mod(y,2*pi);

== matlab function foc_signum_smo_g4/Sliding Mode Observer/SMO bemf estimator3/Sigmoid/sigmoid ==
  data: y output; u input; a input
function y = sigmoid(u,a)
% Sigmoid function instead of signum

y = (2/(1+exp(-a*u)))-1;

== matlab function foc_signum_smo_g4/Sliding Mode Observer/SMO bemf estimator3/Sigmoid/sigmoid1 ==
  data: y output; u input; a input
function y = sigmoid(u,a)
% Sigmoid function instead of signum

y = (2/(1+exp(-a*u)))-1;

== matlab function foc_signum_smo_g4/Sliding Mode Observer/SMO bemf estimator1/Sigmoid/sigmoid ==
  data: y output; u input; a input
function y = sigmoid(u,a)
% Sigmoid function instead of signum

y = (2/(1+exp(-a*u)))-1;

== matlab function foc_signum_smo_g4/Sliding Mode Observer/SMO bemf estimator1/Sigmoid/sigmoid1 ==
  data: y output; u input; a input
function y = sigmoid(u,a)
% Sigmoid function instead of signum

y = (2/(1+exp(-a*u)))-1;

== matlab function foc_signum_smo_g4/Motor model/normalize angle ==
  data: u input; y output
function y = norm_angle(u)
% Normalize angle in radians to between -pi and pi using Matlab's
% wraptopi()

y = wrapToPi(u);
